simulink model "pll_mod"  (R2022b)
settings: Solver=FixedStepDiscrete  StartTime=0.0  StopTime=10  FixedStep=4e-6  RelTol=1e-3
InitFcn:
  | compile;
settings Model: Creator=76475  LastModifiedBy=76475

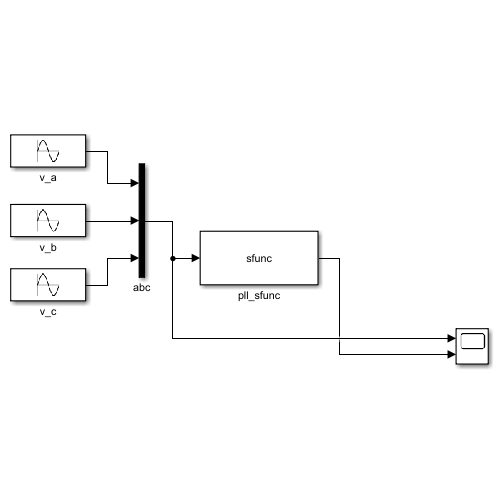
[thumbnail: Simulink's stored preview of the top-level diagram]
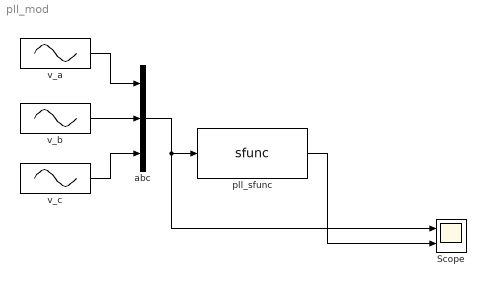
== system pll_mod ==
  Scope : Scope  NumInputPorts=2
  abc : Mux  Inputs=3
  pll_sfunc : S-Function  FunctionName=sfunc  SFunctionDeploymentMode=off  EnableBusSupport=off
  v_a : Sin  Amplitude=34.5e3*sqrt(2)  Frequency=2*pi*50  Phase=pi/2  SampleTime=0
  v_b : Sin  Amplitude=34.5e3*sqrt(2)  Frequency=2*pi*50  Phase=pi/2 - 2*pi/3  SampleTime=0
  v_c : Sin  Amplitude=34.5e3*sqrt(2)  Frequency=2*pi*50  Phase=pi/2 + 2*pi/3  SampleTime=0
  wires:
  v_a/1 -> abc/1
  v_b/1 -> abc/2
  pll_sfunc/1 -> Scope/2
  v_c/1 -> abc/3
  abc/1 -> Scope/1, pll_sfunc/1
